simulink model "ME565_Simulation2_QuarterCar_Linear"  (R2025b)
settings: Solver=VariableStepAuto  StartTime=0.0  StopTime=10.0  RelTol=1e-3
undefined symbols (not defined in the file): Cs, Ct, Ks, Kt, ms, mu

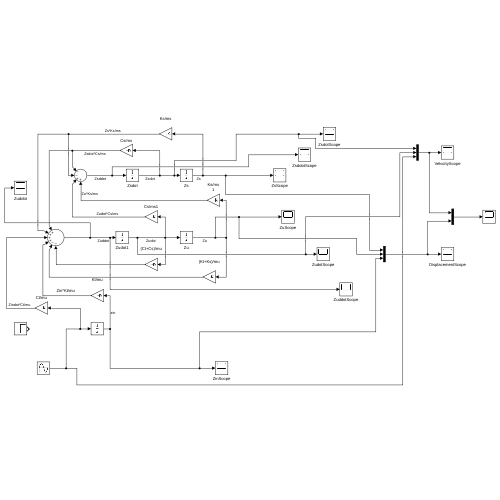
[thumbnail: Simulink's stored preview of the top-level diagram]
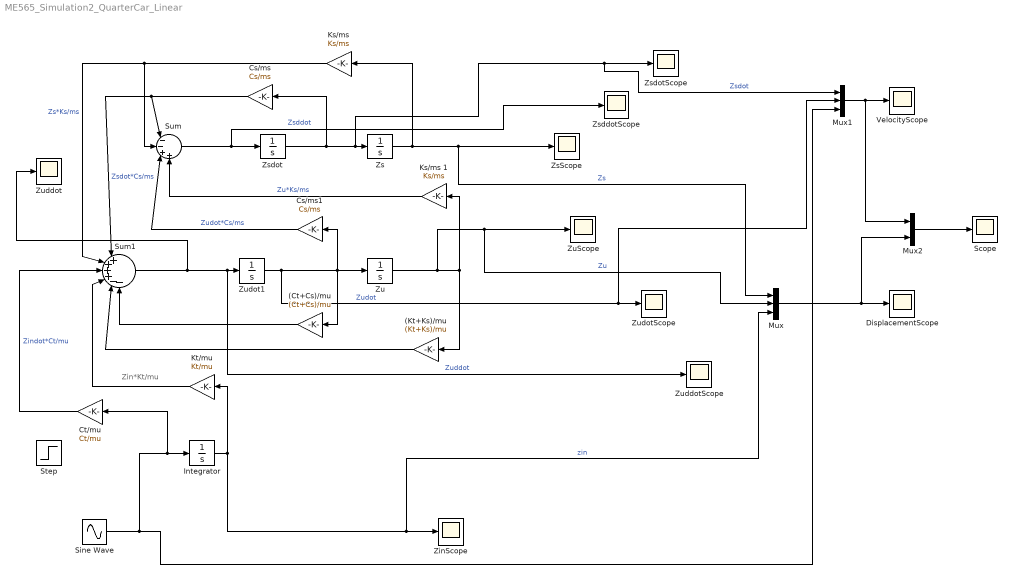
== system ME565_Simulation2_QuarterCar_Linear ==
  note: Zin*Kt/mu
  " Ct/mu" : Gain  Gain=Ct/mu
  "(Ct+Cs)/mu " : Gain  Gain=(Ct+Cs)/mu
  "(Kt+Ks)/mu " : Gain  Gain=(Kt+Ks)/mu
  Cs/ms : Gain  Gain=Cs/ms
  Cs/ms1 : Gain  Gain=Cs/ms
  DisplacementScope : Scope
      settings: ActiveDisplayYMinimum=-0.15421762279986728  ActiveDisplayYMaximum=2.1845765790379228  DataLoggingVariableName=ScopeData8
  Integrator : Integrator
  "Ks/ms " : Gain  Gain=Ks/ms
  Ks/ms 1 : Gain  Gain=Ks/ms
  "Kt/mu " : Gain  Gain=Kt/mu
  Mux : Mux  Inputs=3
  Mux1 : Mux  Inputs=3
  Mux2 : Mux  Inputs=2
  Scope : Scope
      settings: ActiveDisplayYMinimum=-2.8920795092447715  ActiveDisplayYMaximum=3.5208785880839697  DataLoggingVariableName=ScopeData10
  Sine Wave : Sin  SampleTime=0
  Step : Step  After=0.1  SampleTime=0
  Sum : Sum  Inputs=|--++
  Sum1 : Sum  Inputs=|++++--
  VelocityScope : Scope
      settings: ActiveDisplayYMinimum=-0.66532210019380345  ActiveDisplayYMaximum=2.9535851586777206  DataLoggingVariableName=ScopeData9
  ZinScope : Scope
      settings: ActiveDisplayYMinimum=-0.24997835585428682  ActiveDisplayYMaximum=2.2498052026885818  DataLoggingVariableName=ScopeData7
  Zs : Integrator
  ZsScope : Scope
      settings: ActiveDisplayYMinimum=-0.13355062818085633  ActiveDisplayYMaximum=0.86016503882013617  DataLoggingVariableName=ScopeData6
  ZsddotScope : Scope
      settings: ActiveDisplayYMinimum=-0.13355062818085633  ActiveDisplayYMaximum=0.86016503882013617
  Zsdot : Integrator
  ZsdotScope : Scope
      settings: ActiveDisplayYMinimum=-0.013200835443351112  ActiveDisplayYMaximum=0.11880751899016004  DataLoggingVariableName=ScopeData2
  Zu : Integrator
  ZuScope : Scope
      settings: ActiveDisplayYMinimum=-0.13355062818085633  ActiveDisplayYMaximum=0.86016503882013617  DataLoggingVariableName=ScopeData5
  Zuddot : Scope
      settings: ActiveDisplayYMinimum=-0.3257653014204045  ActiveDisplayYMaximum=2.6600115422280761
  ZuddotScope : Scope
      settings: ActiveDisplayYMinimum=-0.13355062818085633  ActiveDisplayYMaximum=0.86016503882013617  DataLoggingVariableName=ScopeData3
  Zudot1 : Integrator
  ZudotScope : Scope
      settings: ActiveDisplayYMinimum=-0.13355062818085633  ActiveDisplayYMaximum=0.86016503882013617  DataLoggingVariableName=ScopeData4
  wires:
  Zsdot/1 -> Cs/ms/1, Mux1/1, ZsdotScope/1, Zs/1  "Zsdot"
  Sum/1 -> ZsddotScope/1, Zsdot/1  "Zsddot"
  Zudot1/1 -> Zu/1, "(Ct+Cs)/mu "/1, Cs/ms1/1, Mux1/2, ZudotScope/1  "Zudot"
  Sum1/1 -> ZuddotScope/1, Zudot1/1, Zuddot/1  "Zuddot"
  Zs/1 -> Mux/1, ZsScope/1, "Ks/ms "/1  "Zs"
  Zu/1 -> Mux/2, ZuScope/1, "(Kt+Ks)/mu "/1, Ks/ms 1/1  "Zu"
  "Ks/ms "/1 -> Sum1/2, Sum/2  "Zs*Ks/ms"
  Cs/ms/1 -> Sum/1, Sum1/1  "Zsdot*Cs/ms"
  Ks/ms 1/1 -> Sum/4  "Zu*Ks/ms"
  Cs/ms1/1 -> Sum/3  "Zudot*Cs/ms"
  "(Ct+Cs)/mu "/1 -> Sum1/6
  "(Kt+Ks)/mu "/1 -> Sum1/5
  Integrator/1 -> "Kt/mu "/1, Mux/3, ZinScope/1  "zin"
  " Ct/mu"/1 -> Sum1/3  "Zindot*Ct/mu"
  "Kt/mu "/1 -> Sum1/4
  Sine Wave/1 -> Mux1/3, " Ct/mu"/1, Integrator/1
  Mux1/1 -> Mux2/1, VelocityScope/1
  Mux/1 -> Mux2/2, DisplacementScope/1
  Mux2/1 -> Scope/1
